simulink model "simulinkOdom"  (R2021b)
settings: Solver=VariableStepAuto  StartTime=0.0  StopTime=10.0  RelTol=1e-3
settings Model: Creator=sanpo  LastModifiedBy=sanpo

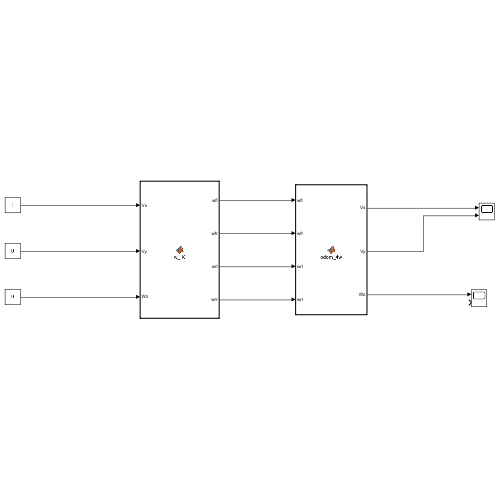
[thumbnail: Simulink's stored preview of the top-level diagram]
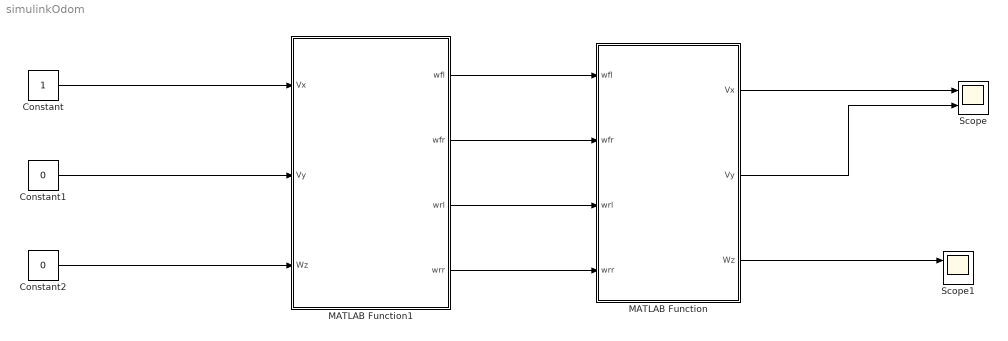
== system simulinkOdom ==
  Constant : Constant
  Constant1 : Constant  Value=0
  Constant2 : Constant  Value=0
  MATLAB Function : MATLAB Function  TreatAsAtomicUnit=on
  MATLAB Function1 : MATLAB Function  TreatAsAtomicUnit=on
  Scope : Scope  NumInputPorts=2
  Scope1 : Scope  NumInputPorts=2
  wires:
  MATLAB Function/1(Vx) -> Scope/1
  MATLAB Function/2(Vy) -> Scope/2
  MATLAB Function/3(Wz) -> Scope1/1
  MATLAB Function1/1(wfl) -> MATLAB Function/1(wfl)
  MATLAB Function1/2(wfr) -> MATLAB Function/2(wfr)
  MATLAB Function1/3(wrl) -> MATLAB Function/3(wrl)
  MATLAB Function1/4(wrr) -> MATLAB Function/4(wrr)
  Constant/1 -> MATLAB Function1/1(Vx)
  Constant1/1 -> MATLAB Function1/2(Vy)
  Constant2/1 -> MATLAB Function1/3(Wz)

== matlab function simulinkOdom/MATLAB Function1 ==
  data: Vx input; wfl output; wfr output; wrl output; wrr output; Vy input; Wz input
function [wfl,wfr,wrl,wrr] =  w_IK(Vx,Vy,Wz)

r = 1;
lx = 1;
ly = 1;
%---------------------
J = [1 -1 -(lx+ly);
    1 1 (lx+ly);
    1 1 -(lx+ly);
    1 -1 (lx+ly)]
W = (1/r)*J*[Vx;Vy;Wz];

wfl = W(1);
wfr = W(2);
wrl = W(3);
wrr = W(4);

== matlab function simulinkOdom/MATLAB Function ==
  data: wfl input; Vx output; wfr input; wrl input; wrr input; Vy output; Wz output

function [Vx,Vy,Wz] = odom_4w(wfl,wfr,wrl,wrr)
%-------------------
r = 1;
lx = 1;
ly = 1;
%---------------------
V = (r/4)*[1 1 1 1;
          -1 1 1 -1;
          -(1/(lx+ly)) (1/(lx+ly)) -(1/(lx+ly)) (1/(lx+ly))]*[wfl;wfr;wrl;wrr];
Vx = V(1);
Vy = V(2);
Wz = V(3);
end
